simulink model "HubDepotModel"  (Simulink 7.9)
settings: Solver=VariableStepDiscrete  StartTime=0.0  StopTime=100.0  RelTol=1e-3
undefined symbols (not defined in the file or in its folder): CustomerBase_1
libraries: simeventslib x10
(part 1 of 4)
settings Model: Creator=tsprock3  LastModifiedBy=tsprock3
settings DebuggingCC: SimStateOlderReleaseMsg=warning

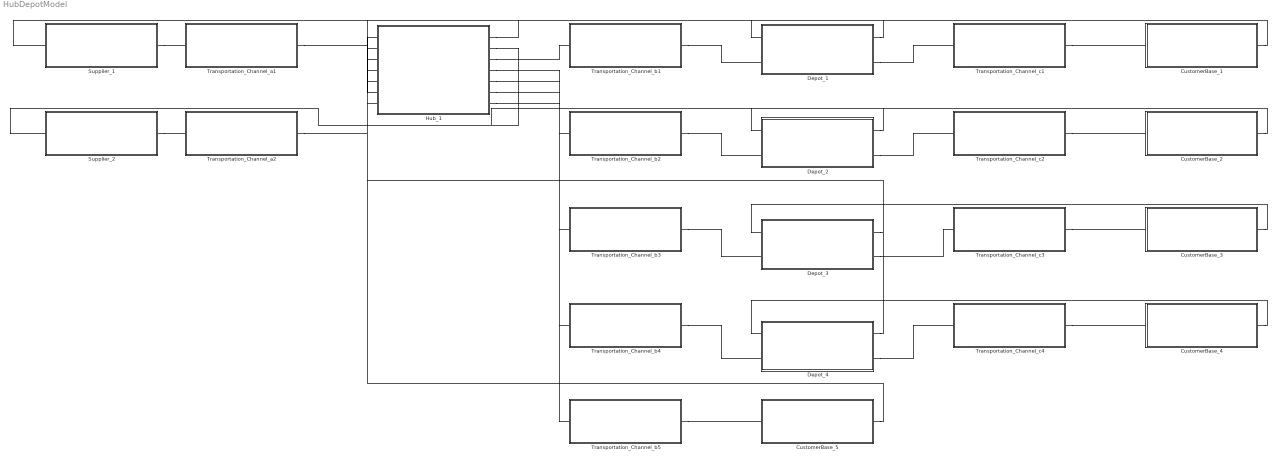
== system HubDepotModel ==
  CustomerBase_1 : Subsystem
  CustomerBase_2 : Subsystem
  CustomerBase_3 : Subsystem
  CustomerBase_4 : Subsystem
  CustomerBase_5 : Subsystem
  Depot_1 : Subsystem
  Depot_2 : Subsystem
  Depot_3 : Subsystem
  Depot_4 : Subsystem
  Hub_1 : Subsystem
  Supplier_1 : Subsystem
  Supplier_2 : Subsystem
  Transportation_Channel_a1 : Subsystem
  Transportation_Channel_a2 : Subsystem
  Transportation_Channel_b1 : Subsystem
  Transportation_Channel_b2 : Subsystem
  Transportation_Channel_b3 : Subsystem
  Transportation_Channel_b4 : Subsystem
  Transportation_Channel_b5 : Subsystem
  Transportation_Channel_c1 : Subsystem
  Transportation_Channel_c2 : Subsystem
  Transportation_Channel_c3 : Subsystem
  Transportation_Channel_c4 : Subsystem
  connections:
  CustomerBase_1/RConn1 -- Depot_1/LConn1
  CustomerBase_2/RConn1 -- Depot_2/LConn1
  CustomerBase_3/RConn1 -- Depot_3/LConn1
  CustomerBase_4/RConn1 -- Depot_4/LConn1
  CustomerBase_5/RConn1 -- Hub_1/LConn1
  Depot_1/RConn1 -- Hub_1/LConn2
  Depot_2/RConn1 -- Hub_1/LConn3
  Depot_3/RConn1 -- Hub_1/LConn4
  Depot_4/RConn1 -- Hub_1/LConn5
  Hub_1/RConn1 -- Supplier_1/LConn1
  Hub_1/RConn2 -- Supplier_2/LConn1
  Supplier_1/RConn1 -- Transportation_Channel_a1/LConn1
  Supplier_2/RConn1 -- Transportation_Channel_a2/LConn1
  Transportation_Channel_a1/RConn1 -- Hub_1/LConn6
  Transportation_Channel_a2/RConn1 -- Hub_1/LConn7
  Hub_1/RConn3 -- Transportation_Channel_b1/LConn1
  Hub_1/RConn4 -- Transportation_Channel_b2/LConn1
  Hub_1/RConn5 -- Transportation_Channel_b3/LConn1
  Hub_1/RConn6 -- Transportation_Channel_b4/LConn1
  Hub_1/RConn7 -- Transportation_Channel_b5/LConn1
  Transportation_Channel_b1/RConn1 -- Depot_1/LConn2
  Transportation_Channel_b2/RConn1 -- Depot_2/LConn2
  Transportation_Channel_b3/RConn1 -- Depot_3/LConn2
  Transportation_Channel_b4/RConn1 -- Depot_4/LConn2
  Depot_1/RConn2 -- Transportation_Channel_c1/LConn1
  Depot_2/RConn2 -- Transportation_Channel_c2/LConn1
  Depot_3/RConn2 -- Transportation_Channel_c3/LConn1
  Depot_4/RConn2 -- Transportation_Channel_c4/LConn1
  Transportation_Channel_b5/RConn1 -- CustomerBase_5/LConn1
  Transportation_Channel_c1/RConn1 -- CustomerBase_1/LConn1
  Transportation_Channel_c2/RConn1 -- CustomerBase_2/LConn1
  Transportation_Channel_c3/RConn1 -- CustomerBase_3/LConn1
  Transportation_Channel_c4/RConn1 -- CustomerBase_4/LConn1

== system HubDepotModel/CustomerBase_1 ==
  CustomerBase : Subsystem
  IN_Shipment : PathCombiner  NumberInputPorts=1
  OUT_Order : OutputSwitch  NumberOutputPorts=1  SwitchingCriterion=From attribute  AttributeName=Supplier
  IN_Shipment_1 : PMIOPort  Port=1  Side=Left
  OUT_Order_1 : PMIOPort  Port=2  Side=Right
  connections:
  IN_Shipment/RConn1 -- CustomerBase/LConn2
  OUT_Order/LConn1 -- CustomerBase/LConn1
  IN_Shipment/LConn1 -- IN_Shipment_1/RConn1
  OUT_Order/RConn1 -- OUT_Order_1/RConn1

== system HubDepotModel/CustomerBase_2 ==
  CustomerBase : Subsystem
  IN_Shipment : PathCombiner  NumberInputPorts=1
  OUT_Order : OutputSwitch  NumberOutputPorts=1  SwitchingCriterion=From attribute  AttributeName=Supplier
  IN_Shipment_1 : PMIOPort  Port=1  Side=Left
  OUT_Order_1 : PMIOPort  Port=2  Side=Right
  connections:
  IN_Shipment/RConn1 -- CustomerBase/LConn2
  OUT_Order/LConn1 -- CustomerBase/LConn1
  IN_Shipment/LConn1 -- IN_Shipment_1/RConn1
  OUT_Order/RConn1 -- OUT_Order_1/RConn1

== system HubDepotModel/CustomerBase_3 ==
  CustomerBase : Subsystem
  IN_Shipment : PathCombiner  NumberInputPorts=1
  OUT_Order : OutputSwitch  NumberOutputPorts=1  SwitchingCriterion=From attribute  AttributeName=Supplier
  IN_Shipment_1 : PMIOPort  Port=1  Side=Left
  OUT_Order_1 : PMIOPort  Port=2  Side=Right
  connections:
  IN_Shipment/RConn1 -- CustomerBase/LConn2
  OUT_Order/LConn1 -- CustomerBase/LConn1
  IN_Shipment/LConn1 -- IN_Shipment_1/RConn1
  OUT_Order/RConn1 -- OUT_Order_1/RConn1

== system HubDepotModel/CustomerBase_4 ==
  CustomerBase : Subsystem
  IN_Shipment : PathCombiner  NumberInputPorts=1
  OUT_Order : OutputSwitch  NumberOutputPorts=1  SwitchingCriterion=From attribute  AttributeName=Supplier
  IN_Shipment_1 : PMIOPort  Port=1  Side=Left
  OUT_Order_1 : PMIOPort  Port=2  Side=Right
  connections:
  IN_Shipment/RConn1 -- CustomerBase/LConn2
  OUT_Order/LConn1 -- CustomerBase/LConn1
  IN_Shipment/LConn1 -- IN_Shipment_1/RConn1
  OUT_Order/RConn1 -- OUT_Order_1/RConn1

== system HubDepotModel/CustomerBase_5 ==
  CustomerBase : Subsystem
  IN_Shipment : PathCombiner  NumberInputPorts=1
  OUT_Order : OutputSwitch  NumberOutputPorts=1  SwitchingCriterion=From attribute  AttributeName=Supplier
  IN_Shipment_1 : PMIOPort  Port=1  Side=Left
  OUT_Order_1 : PMIOPort  Port=2  Side=Right
  connections:
  IN_Shipment/RConn1 -- CustomerBase/LConn2
  OUT_Order/LConn1 -- CustomerBase/LConn1
  IN_Shipment/LConn1 -- IN_Shipment_1/RConn1
  OUT_Order/RConn1 -- OUT_Order_1/RConn1

== system HubDepotModel/Depot_1 ==
  note: IN_Order
  IN_Order : PathCombiner  NumberInputPorts=1
  IN_Shipment : PathCombiner  NumberInputPorts=1
  OUT_Order : OutputSwitch  NumberOutputPorts=1  SwitchingCriterion=From attribute  AttributeName=Supplier
  OUT_Shipment : OutputSwitch  NumberOutputPorts=1  SwitchingCriterion=From attribute  AttributeName=Customer
  Storage_Subsystem : Subsystem
  IN_Order_1 : PMIOPort  Port=1  Side=Left
  IN_Shipment_1 : PMIOPort  Port=2  Side=Left
  OUT_Order_1 : PMIOPort  Port=3  Side=Right
  OUT_Shipment_1 : PMIOPort  Port=4  Side=Right
  connections:
  Storage_Subsystem/RConn2 -- OUT_Shipment/LConn1
  IN_Order/RConn1 -- Storage_Subsystem/RConn1
  OUT_Order/LConn1 -- Storage_Subsystem/LConn1
  IN_Shipment/RConn1 -- Storage_Subsystem/LConn2
  IN_Order/LConn1 -- IN_Order_1/RConn1
  IN_Shipment/LConn1 -- IN_Shipment_1/RConn1
  OUT_Order/RConn1 -- OUT_Order_1/RConn1
  OUT_Shipment/RConn1 -- OUT_Shipment_1/RConn1

== system HubDepotModel/Depot_2 ==
  note: IN_Order
  IN_Order : PathCombiner  NumberInputPorts=1
  IN_Shipment : PathCombiner  NumberInputPorts=1
  OUT_Order : OutputSwitch  NumberOutputPorts=1  SwitchingCriterion=From attribute  AttributeName=Supplier
  OUT_Shipment : OutputSwitch  NumberOutputPorts=1  SwitchingCriterion=From attribute  AttributeName=Customer
  Storage_Subsystem : Subsystem
  IN_Order_1 : PMIOPort  Port=1  Side=Left
  IN_Shipment_1 : PMIOPort  Port=2  Side=Left
  OUT_Order_1 : PMIOPort  Port=3  Side=Right
  OUT_Shipment_1 : PMIOPort  Port=4  Side=Right
  connections:
  Storage_Subsystem/RConn2 -- OUT_Shipment/LConn1
  IN_Order/RConn1 -- Storage_Subsystem/RConn1
  OUT_Order/LConn1 -- Storage_Subsystem/LConn1
  IN_Shipment/RConn1 -- Storage_Subsystem/LConn2
  IN_Order/LConn1 -- IN_Order_1/RConn1
  IN_Shipment/LConn1 -- IN_Shipment_1/RConn1
  OUT_Order/RConn1 -- OUT_Order_1/RConn1
  OUT_Shipment/RConn1 -- OUT_Shipment_1/RConn1

== system HubDepotModel/Depot_3 ==
  note: IN_Order
  IN_Order : PathCombiner  NumberInputPorts=1
  IN_Shipment : PathCombiner  NumberInputPorts=1
  OUT_Order : OutputSwitch  NumberOutputPorts=1  SwitchingCriterion=From attribute  AttributeName=Supplier
  OUT_Shipment : OutputSwitch  NumberOutputPorts=1  SwitchingCriterion=From attribute  AttributeName=Customer
  Storage_Subsystem : Subsystem
  IN_Order_1 : PMIOPort  Port=1  Side=Left
  IN_Shipment_1 : PMIOPort  Port=2  Side=Left
  OUT_Order_1 : PMIOPort  Port=3  Side=Right
  OUT_Shipment_1 : PMIOPort  Port=4  Side=Right
  connections:
  Storage_Subsystem/RConn2 -- OUT_Shipment/LConn1
  IN_Order/RConn1 -- Storage_Subsystem/RConn1
  OUT_Order/LConn1 -- Storage_Subsystem/LConn1
  IN_Shipment/RConn1 -- Storage_Subsystem/LConn2
  IN_Order/LConn1 -- IN_Order_1/RConn1
  IN_Shipment/LConn1 -- IN_Shipment_1/RConn1
  OUT_Order/RConn1 -- OUT_Order_1/RConn1
  OUT_Shipment/RConn1 -- OUT_Shipment_1/RConn1

== system HubDepotModel/Depot_4 ==
  note: IN_Order
  IN_Order : PathCombiner  NumberInputPorts=1
  IN_Shipment : PathCombiner  NumberInputPorts=1
  OUT_Order : OutputSwitch  NumberOutputPorts=1  SwitchingCriterion=From attribute  AttributeName=Supplier
  OUT_Shipment : OutputSwitch  NumberOutputPorts=1  SwitchingCriterion=From attribute  AttributeName=Customer
  Storage_Subsystem : Subsystem
  IN_Order_1 : PMIOPort  Port=1  Side=Left
  IN_Shipment_1 : PMIOPort  Port=2  Side=Left
  OUT_Order_1 : PMIOPort  Port=3  Side=Right
  OUT_Shipment_1 : PMIOPort  Port=4  Side=Right
  connections:
  Storage_Subsystem/RConn2 -- OUT_Shipment/LConn1
  IN_Order/RConn1 -- Storage_Subsystem/RConn1
  OUT_Order/LConn1 -- Storage_Subsystem/LConn1
  IN_Shipment/RConn1 -- Storage_Subsystem/LConn2
  IN_Order/LConn1 -- IN_Order_1/RConn1
  IN_Shipment/LConn1 -- IN_Shipment_1/RConn1
  OUT_Order/RConn1 -- OUT_Order_1/RConn1
  OUT_Shipment/RConn1 -- OUT_Shipment_1/RConn1

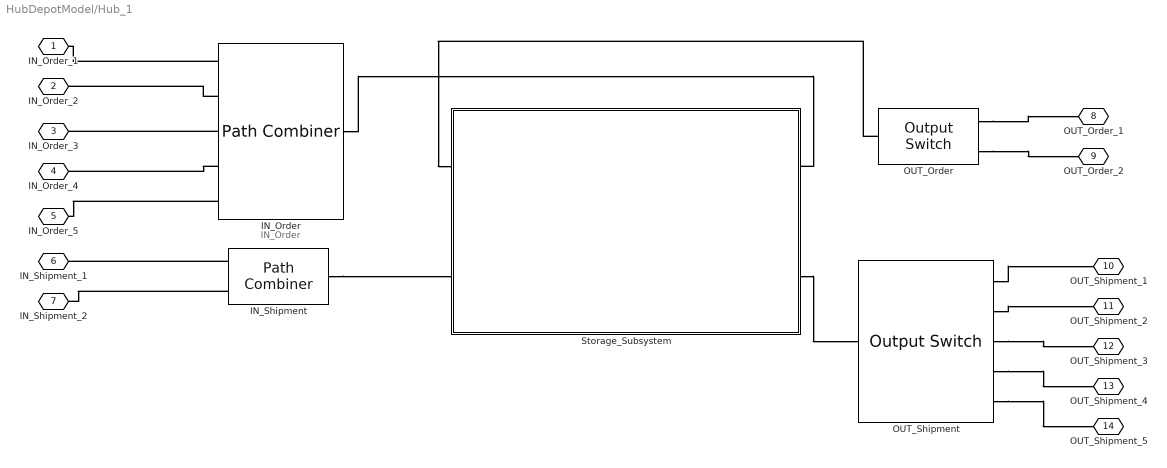
== system HubDepotModel/Hub_1 ==
  note: IN_Order
  IN_Order : PathCombiner  NumberInputPorts=5
  IN_Shipment : PathCombiner  NumberInputPorts=2
  OUT_Order : OutputSwitch  NumberOutputPorts=2  SwitchingCriterion=From attribute  AttributeName=Supplier
  OUT_Shipment : OutputSwitch  NumberOutputPorts=5  SwitchingCriterion=From attribute  AttributeName=Customer
  Storage_Subsystem : Subsystem
  IN_Order_1 : PMIOPort  Port=1  Side=Left
  IN_Order_2 : PMIOPort  Port=2  Side=Left
  IN_Order_3 : PMIOPort  Port=3  Side=Left
  IN_Order_4 : PMIOPort  Port=4  Side=Left
  IN_Order_5 : PMIOPort  Port=5  Side=Left
  IN_Shipment_1 : PMIOPort  Port=6  Side=Left
  IN_Shipment_2 : PMIOPort  Port=7  Side=Left
  OUT_Order_1 : PMIOPort  Port=8  Side=Right
  OUT_Order_2 : PMIOPort  Port=9  Side=Right
  OUT_Shipment_1 : PMIOPort  Port=10  Side=Right
  OUT_Shipment_2 : PMIOPort  Port=11  Side=Right
  OUT_Shipment_3 : PMIOPort  Port=12  Side=Right
  OUT_Shipment_4 : PMIOPort  Port=13  Side=Right
  OUT_Shipment_5 : PMIOPort  Port=14  Side=Right
  connections:
  Storage_Subsystem/RConn2 -- OUT_Shipment/LConn1
  IN_Order/RConn1 -- Storage_Subsystem/RConn1
  OUT_Order/LConn1 -- Storage_Subsystem/LConn1
  IN_Shipment/RConn1 -- Storage_Subsystem/LConn2
  IN_Order/LConn1 -- IN_Order_1/RConn1
  IN_Order/LConn2 -- IN_Order_2/RConn1
  IN_Order/LConn3 -- IN_Order_3/RConn1
  IN_Order/LConn4 -- IN_Order_4/RConn1
  IN_Order/LConn5 -- IN_Order_5/RConn1
  IN_Shipment/LConn1 -- IN_Shipment_1/RConn1
  IN_Shipment/LConn2 -- IN_Shipment_2/RConn1
  OUT_Order/RConn1 -- OUT_Order_1/RConn1
  OUT_Order/RConn2 -- OUT_Order_2/RConn1
  OUT_Shipment/RConn1 -- OUT_Shipment_1/RConn1
  OUT_Shipment/RConn2 -- OUT_Shipment_2/RConn1
  OUT_Shipment/RConn3 -- OUT_Shipment_3/RConn1
  OUT_Shipment/RConn4 -- OUT_Shipment_4/RConn1
  OUT_Shipment/RConn5 -- OUT_Shipment_5/RConn1

== system HubDepotModel/Supplier_1 ==
  IN_Order : PathCombiner  NumberInputPorts=1
  OUT_Shipment : OutputSwitch  NumberOutputPorts=1  SwitchingCriterion=From attribute  AttributeName=Customer
  Supplier : Subsystem
  IN_Order_1 : PMIOPort  Port=1  Side=Left
  OUT_Shipment_1 : PMIOPort  Port=2  Side=Right
  connections:
  IN_Order/RConn1 -- Supplier/RConn2
  OUT_Shipment/LConn1 -- Supplier/RConn1
  IN_Order/LConn1 -- IN_Order_1/RConn1
  OUT_Shipment/RConn1 -- OUT_Shipment_1/RConn1

== system HubDepotModel/Supplier_2 ==
  IN_Order : PathCombiner  NumberInputPorts=1
  OUT_Shipment : OutputSwitch  NumberOutputPorts=1  SwitchingCriterion=From attribute  AttributeName=Customer
  Supplier : Subsystem
  IN_Order_1 : PMIOPort  Port=1  Side=Left
  OUT_Shipment_1 : PMIOPort  Port=2  Side=Right
  connections:
  IN_Order/RConn1 -- Supplier/RConn2
  OUT_Shipment/LConn1 -- Supplier/RConn1
  IN_Order/LConn1 -- IN_Order_1/RConn1
  OUT_Shipment/RConn1 -- OUT_Shipment_1/RConn1

== system HubDepotModel/Transportation_Channel_a1 ==
  FIFO Queue : FIFOQueue  Capacity=inf
  IN_Shipment : PathCombiner  NumberInputPorts=1
  N-Server : NServer  NumberOfServers=inf  ServiceTime=0
  OUT_Shipment : OutputSwitch  NumberOutputPorts=1  AttributeName=Customer
  IN_Shipment_1 : PMIOPort  Port=1  Side=Left
  OUT_Shipment_1 : PMIOPort  Port=2  Side=Right
  connections:
  N-Server/RConn1 -- OUT_Shipment/LConn1
  IN_Shipment/RConn1 -- FIFO Queue/LConn1
  FIFO Queue/RConn1 -- N-Server/LConn1
  IN_Shipment/LConn1 -- IN_Shipment_1/RConn1
  OUT_Shipment/RConn1 -- OUT_Shipment_1/RConn1

== system HubDepotModel/Transportation_Channel_a2 ==
  FIFO Queue : FIFOQueue  Capacity=inf
  IN_Shipment : PathCombiner  NumberInputPorts=1
  N-Server : NServer  NumberOfServers=inf  ServiceTime=0
  OUT_Shipment : OutputSwitch  NumberOutputPorts=1  AttributeName=Customer
  IN_Shipment_1 : PMIOPort  Port=1  Side=Left
  OUT_Shipment_1 : PMIOPort  Port=2  Side=Right
  connections:
  N-Server/RConn1 -- OUT_Shipment/LConn1
  IN_Shipment/RConn1 -- FIFO Queue/LConn1
  FIFO Queue/RConn1 -- N-Server/LConn1
  IN_Shipment/LConn1 -- IN_Shipment_1/RConn1
  OUT_Shipment/RConn1 -- OUT_Shipment_1/RConn1

== system HubDepotModel/Transportation_Channel_b1 ==
  FIFO Queue : FIFOQueue  Capacity=inf
  IN_Shipment : PathCombiner  NumberInputPorts=1
  N-Server : NServer  NumberOfServers=inf  ServiceTime=0
  OUT_Shipment : OutputSwitch  NumberOutputPorts=1  AttributeName=Customer
  IN_Shipment_1 : PMIOPort  Port=1  Side=Left
  OUT_Shipment_1 : PMIOPort  Port=2  Side=Right
  connections:
  N-Server/RConn1 -- OUT_Shipment/LConn1
  IN_Shipment/RConn1 -- FIFO Queue/LConn1
  FIFO Queue/RConn1 -- N-Server/LConn1
  IN_Shipment/LConn1 -- IN_Shipment_1/RConn1
  OUT_Shipment/RConn1 -- OUT_Shipment_1/RConn1

== system HubDepotModel/Transportation_Channel_b2 ==
  FIFO Queue : FIFOQueue  Capacity=inf
  IN_Shipment : PathCombiner  NumberInputPorts=1
  N-Server : NServer  NumberOfServers=inf  ServiceTime=0
  OUT_Shipment : OutputSwitch  NumberOutputPorts=1  AttributeName=Customer
  IN_Shipment_1 : PMIOPort  Port=1  Side=Left
  OUT_Shipment_1 : PMIOPort  Port=2  Side=Right
  connections:
  N-Server/RConn1 -- OUT_Shipment/LConn1
  IN_Shipment/RConn1 -- FIFO Queue/LConn1
  FIFO Queue/RConn1 -- N-Server/LConn1
  IN_Shipment/LConn1 -- IN_Shipment_1/RConn1
  OUT_Shipment/RConn1 -- OUT_Shipment_1/RConn1

== system HubDepotModel/Transportation_Channel_b3 ==
  FIFO Queue : FIFOQueue  Capacity=inf
  IN_Shipment : PathCombiner  NumberInputPorts=1
  N-Server : NServer  NumberOfServers=inf  ServiceTime=0
  OUT_Shipment : OutputSwitch  NumberOutputPorts=1  AttributeName=Customer
  IN_Shipment_1 : PMIOPort  Port=1  Side=Left
  OUT_Shipment_1 : PMIOPort  Port=2  Side=Right
  connections:
  N-Server/RConn1 -- OUT_Shipment/LConn1
  IN_Shipment/RConn1 -- FIFO Queue/LConn1
  FIFO Queue/RConn1 -- N-Server/LConn1
  IN_Shipment/LConn1 -- IN_Shipment_1/RConn1
  OUT_Shipment/RConn1 -- OUT_Shipment_1/RConn1

== system HubDepotModel/Transportation_Channel_b4 ==
  FIFO Queue : FIFOQueue  Capacity=inf
  IN_Shipment : PathCombiner  NumberInputPorts=1
  N-Server : NServer  NumberOfServers=inf  ServiceTime=0
  OUT_Shipment : OutputSwitch  NumberOutputPorts=1  AttributeName=Customer
  IN_Shipment_1 : PMIOPort  Port=1  Side=Left
  OUT_Shipment_1 : PMIOPort  Port=2  Side=Right
  connections:
  N-Server/RConn1 -- OUT_Shipment/LConn1
  IN_Shipment/RConn1 -- FIFO Queue/LConn1
  FIFO Queue/RConn1 -- N-Server/LConn1
  IN_Shipment/LConn1 -- IN_Shipment_1/RConn1
  OUT_Shipment/RConn1 -- OUT_Shipment_1/RConn1

== system HubDepotModel/Transportation_Channel_b5 ==
  FIFO Queue : FIFOQueue  Capacity=inf
  IN_Shipment : PathCombiner  NumberInputPorts=1
  N-Server : NServer  NumberOfServers=inf  ServiceTime=0
  OUT_Shipment : OutputSwitch  NumberOutputPorts=1  AttributeName=Customer
  IN_Shipment_1 : PMIOPort  Port=1  Side=Left
  OUT_Shipment_1 : PMIOPort  Port=2  Side=Right
  connections:
  N-Server/RConn1 -- OUT_Shipment/LConn1
  IN_Shipment/RConn1 -- FIFO Queue/LConn1
  FIFO Queue/RConn1 -- N-Server/LConn1
  IN_Shipment/LConn1 -- IN_Shipment_1/RConn1
  OUT_Shipment/RConn1 -- OUT_Shipment_1/RConn1

== system HubDepotModel/Transportation_Channel_c1 ==
  FIFO Queue : FIFOQueue  Capacity=inf
  IN_Shipment : PathCombiner  NumberInputPorts=1
  N-Server : NServer  NumberOfServers=inf  ServiceTime=0
  OUT_Shipment : OutputSwitch  NumberOutputPorts=1  AttributeName=Customer
  IN_Shipment_1 : PMIOPort  Port=1  Side=Left
  OUT_Shipment_1 : PMIOPort  Port=2  Side=Right
  connections:
  N-Server/RConn1 -- OUT_Shipment/LConn1
  IN_Shipment/RConn1 -- FIFO Queue/LConn1
  FIFO Queue/RConn1 -- N-Server/LConn1
  IN_Shipment/LConn1 -- IN_Shipment_1/RConn1
  OUT_Shipment/RConn1 -- OUT_Shipment_1/RConn1

== system HubDepotModel/Transportation_Channel_c2 ==
  FIFO Queue : FIFOQueue  Capacity=inf
  IN_Shipment : PathCombiner  NumberInputPorts=1
  N-Server : NServer  NumberOfServers=inf  ServiceTime=0
  OUT_Shipment : OutputSwitch  NumberOutputPorts=1  AttributeName=Customer
  IN_Shipment_1 : PMIOPort  Port=1  Side=Left
  OUT_Shipment_1 : PMIOPort  Port=2  Side=Right
  connections:
  N-Server/RConn1 -- OUT_Shipment/LConn1
  IN_Shipment/RConn1 -- FIFO Queue/LConn1
  FIFO Queue/RConn1 -- N-Server/LConn1
  IN_Shipment/LConn1 -- IN_Shipment_1/RConn1
  OUT_Shipment/RConn1 -- OUT_Shipment_1/RConn1

== system HubDepotModel/Transportation_Channel_c3 ==
  FIFO Queue : FIFOQueue  Capacity=inf
  IN_Shipment : PathCombiner  NumberInputPorts=1
  N-Server : NServer  NumberOfServers=inf  ServiceTime=0
  OUT_Shipment : OutputSwitch  NumberOutputPorts=1  AttributeName=Customer
  IN_Shipment_1 : PMIOPort  Port=1  Side=Left
  OUT_Shipment_1 : PMIOPort  Port=2  Side=Right
  connections:
  N-Server/RConn1 -- OUT_Shipment/LConn1
  IN_Shipment/RConn1 -- FIFO Queue/LConn1
  FIFO Queue/RConn1 -- N-Server/LConn1
  IN_Shipment/LConn1 -- IN_Shipment_1/RConn1
  OUT_Shipment/RConn1 -- OUT_Shipment_1/RConn1

== system HubDepotModel/Transportation_Channel_c4 ==
  FIFO Queue : FIFOQueue  Capacity=inf
  IN_Shipment : PathCombiner  NumberInputPorts=1
  N-Server : NServer  NumberOfServers=inf  ServiceTime=0
  OUT_Shipment : OutputSwitch  NumberOutputPorts=1  AttributeName=Customer
  IN_Shipment_1 : PMIOPort  Port=1  Side=Left
  OUT_Shipment_1 : PMIOPort  Port=2  Side=Right
  connections:
  N-Server/RConn1 -- OUT_Shipment/LConn1
  IN_Shipment/RConn1 -- FIFO Queue/LConn1
  FIFO Queue/RConn1 -- N-Server/LConn1
  IN_Shipment/LConn1 -- IN_Shipment_1/RConn1
  OUT_Shipment/RConn1 -- OUT_Shipment_1/RConn1

== system HubDepotModel/CustomerBase_1/CustomerBase ==
  Consumption_Component : EventBasedSequence  VectorOutputValues=CustomerBase_1(:,1)
  Entity Sink : EntitySink
  Order_Generator : TimeBasedEntityGenerator  GenerateEntitiesUpon=Intergeneration time from port t  GenerateEntityAtSimulationStart=off
  Order_Quantity : EventBasedSequence  VectorOutputValues=CustomerBase_1(:,2)
  Order_Time : EventBasedSequence  VectorOutputValues=CustomerBase_1(:,3)  FormOutputOpt=Setting to infinity
  Set_Procurement_Order : SetAttribute  AttributeName=Component|Order_Quantity|Customer|Supplier  AttributeFrom=Signal port|Signal port|Dialog|Dialog  AttributeValue=1|3|1|1  AttributeTreatAsVector=1|1|1|1  EvaluatedAttributeValue={[];[];1;1}
      settings: InputPortMap=u0,u1
  Procurement_Order : PMIOPort  Port=1  Side=Left
  Replenishment_Shipment : PMIOPort  Port=2  Side=Left
  wires:
  Consumption_Component/1 -> Set_Procurement_Order/1
  Order_Quantity/1 -> Set_Procurement_Order/2
  Order_Time/1 -> Order_Generator/1
  connections:
  Replenishment_Shipment/RConn1 -- Entity Sink/LConn1
  Procurement_Order/RConn1 -- Set_Procurement_Order/RConn1
  Order_Generator/RConn1 -- Set_Procurement_Order/LConn1

== system HubDepotModel/CustomerBase_2/CustomerBase ==
  Consumption_Component : EventBasedSequence  VectorOutputValues=[2 1 2 1 2 1].'
  Entity Sink : EntitySink
  Order_Generator : TimeBasedEntityGenerator  GenerateEntitiesUpon=Intergeneration time from port t  GenerateEntityAtSimulationStart=off
  Order_Quantity : EventBasedRandomNumber  Distribution=Arbitrary discrete  valueVecDisc=[1 2 3 4 5]  probVecDisc=[0.2 0.2 0.2 0.2 0.2]  Seed=46469
  Order_Time : EventBasedSequence  VectorOutputValues=[0; 0; 1; 0; 1; 1; 1; 0; 0; 1; 1; 0; 1].'
  Set_Procurement_Order : SetAttribute  AttributeName=Component|Order_Quantity|Customer|Supplier  AttributeFrom=Signal port|Signal port|Dialog|Dialog  AttributeValue=1|3|1|1  AttributeTreatAsVector=1|1|1|1  EvaluatedAttributeValue={[];[];1;1}
      settings: InputPortMap=u0,u1
  Procurement_Order : PMIOPort  Port=1  Side=Left
  Replenishment_Shipment : PMIOPort  Port=2  Side=Left
  wires:
  Consumption_Component/1 -> Set_Procurement_Order/1
  Order_Quantity/1 -> Set_Procurement_Order/2
  Order_Time/1 -> Order_Generator/1
  connections:
  Replenishment_Shipment/RConn1 -- Entity Sink/LConn1
  Procurement_Order/RConn1 -- Set_Procurement_Order/RConn1
  Order_Generator/RConn1 -- Set_Procurement_Order/LConn1

== system HubDepotModel/CustomerBase_3/CustomerBase ==
  Consumption_Component : EventBasedSequence  VectorOutputValues=[2 1 2 1 2 1].'
  Entity Sink : EntitySink
  Order_Generator : TimeBasedEntityGenerator  GenerateEntitiesUpon=Intergeneration time from port t  GenerateEntityAtSimulationStart=off
  Order_Quantity : EventBasedRandomNumber  Distribution=Arbitrary discrete  valueVecDisc=[1 2 3 4 5]  probVecDisc=[0.2 0.2 0.2 0.2 0.2]  Seed=1431
  Order_Time : EventBasedSequence  VectorOutputValues=[0; 0; 1; 0; 1; 1; 1; 0; 0; 1; 1; 0; 1].'
  Set_Procurement_Order : SetAttribute  AttributeName=Component|Order_Quantity|Customer|Supplier  AttributeFrom=Signal port|Signal port|Dialog|Dialog  AttributeValue=1|3|1|1  AttributeTreatAsVector=1|1|1|1  EvaluatedAttributeValue={[];[];1;1}
      settings: InputPortMap=u0,u1
  Procurement_Order : PMIOPort  Port=1  Side=Left
  Replenishment_Shipment : PMIOPort  Port=2  Side=Left
  wires:
  Consumption_Component/1 -> Set_Procurement_Order/1
  Order_Quantity/1 -> Set_Procurement_Order/2
  Order_Time/1 -> Order_Generator/1
  connections:
  Replenishment_Shipment/RConn1 -- Entity Sink/LConn1
  Procurement_Order/RConn1 -- Set_Procurement_Order/RConn1
  Order_Generator/RConn1 -- Set_Procurement_Order/LConn1

== system HubDepotModel/CustomerBase_4/CustomerBase ==
  Consumption_Component : EventBasedSequence  VectorOutputValues=[2 1 2 1 2 1].'
  Entity Sink : EntitySink
  Order_Generator : TimeBasedEntityGenerator  GenerateEntitiesUpon=Intergeneration time from port t  GenerateEntityAtSimulationStart=off
  Order_Quantity : EventBasedRandomNumber  Distribution=Arbitrary discrete  valueVecDisc=[1 2 3 4 5]  probVecDisc=[0.2 0.2 0.2 0.2 0.2]  Seed=4648
  Order_Time : EventBasedSequence  VectorOutputValues=[0; 0; 1; 0; 1; 1; 1; 0; 0; 1; 1; 0; 1].'
  Set_Procurement_Order : SetAttribute  AttributeName=Component|Order_Quantity|Customer|Supplier  AttributeFrom=Signal port|Signal port|Dialog|Dialog  AttributeValue=1|3|1|1  AttributeTreatAsVector=1|1|1|1  EvaluatedAttributeValue={[];[];1;1}
      settings: InputPortMap=u0,u1
  Procurement_Order : PMIOPort  Port=1  Side=Left
  Replenishment_Shipment : PMIOPort  Port=2  Side=Left
  wires:
  Consumption_Component/1 -> Set_Procurement_Order/1
  Order_Quantity/1 -> Set_Procurement_Order/2
  Order_Time/1 -> Order_Generator/1
  connections:
  Replenishment_Shipment/RConn1 -- Entity Sink/LConn1
  Procurement_Order/RConn1 -- Set_Procurement_Order/RConn1
  Order_Generator/RConn1 -- Set_Procurement_Order/LConn1

== system HubDepotModel/CustomerBase_5/CustomerBase ==
  Consumption_Component : EventBasedSequence  VectorOutputValues=[2 1 2 1 2 1].'
  Entity Sink : EntitySink
  Order_Generator : TimeBasedEntityGenerator  GenerateEntitiesUpon=Intergeneration time from port t  GenerateEntityAtSimulationStart=off
  Order_Quantity : EventBasedRandomNumber  Distribution=Arbitrary discrete  valueVecDisc=[1 2 3 4 5]  probVecDisc=[0.2 0.2 0.2 0.2 0.2]  Seed=7865
  Order_Time : EventBasedSequence  VectorOutputValues=[0; 0; 1; 0; 1; 1; 1; 0; 0; 1; 1; 0; 1].'
  Set_Procurement_Order : SetAttribute  AttributeName=Component|Order_Quantity|Customer|Supplier  AttributeFrom=Signal port|Signal port|Dialog|Dialog  AttributeValue=1|3|1|1  AttributeTreatAsVector=1|1|1|1  EvaluatedAttributeValue={[];[];1;1}
      settings: InputPortMap=u0,u1
  Procurement_Order : PMIOPort  Port=1  Side=Left
  Replenishment_Shipment : PMIOPort  Port=2  Side=Left
  wires:
  Consumption_Component/1 -> Set_Procurement_Order/1
  Order_Quantity/1 -> Set_Procurement_Order/2
  Order_Time/1 -> Order_Generator/1
  connections:
  Replenishment_Shipment/RConn1 -- Entity Sink/LConn1
  Procurement_Order/RConn1 -- Set_Procurement_Order/RConn1
  Order_Generator/RConn1 -- Set_Procurement_Order/LConn1

== system HubDepotModel/Depot_1/Storage_Subsystem ==
  <<DELIVER>>Deliver_Stocked_Product : Subsystem
  <<ENABLE>> Manage_Product_Inventory : Subsystem
  <<SOURCE>> Source_Stocked_Product : Subsystem
  Customer_Procurement_Order : PMIOPort  Port=1  Side=Right
  Fulfillment_Shipment : PMIOPort  Port=2  Side=Right
  Procurement_Order : PMIOPort  Port=3  Side=Left
  Replenishment_Shipment : PMIOPort  Port=4  Side=Left
  connections:
  <<DELIVER>>Deliver_Stocked_Product/RConn1 -- <<ENABLE>> Manage_Product_Inventory/LConn1
  <<SOURCE>> Source_Stocked_Product/RConn2 -- Procurement_Order/RConn1
  <<ENABLE>> Manage_Product_Inventory/RConn3 -- <<SOURCE>> Source_Stocked_Product/LConn3
  <<ENABLE>> Manage_Product_Inventory/LConn3 -- <<DELIVER>>Deliver_Stocked_Product/RConn3
  <<ENABLE>> Manage_Product_Inventory/RConn2 -- <<SOURCE>> Source_Stocked_Product/LConn1
  <<ENABLE>> Manage_Product_Inventory/LConn2 -- <<SOURCE>> Source_Stocked_Product/RConn1
  Replenishment_Shipment/RConn1 -- <<SOURCE>> Source_Stocked_Product/LConn2
  <<DELIVER>>Deliver_Stocked_Product/RConn2 -- Fulfillment_Shipment/RConn1
  <<DELIVER>>Deliver_Stocked_Product/LConn2 -- Customer_Procurement_Order/RConn1
  <<DELIVER>>Deliver_Stocked_Product/LConn1 -- <<ENABLE>> Manage_Product_Inventory/RConn1

== system HubDepotModel/Depot_2/Storage_Subsystem ==
  <<DELIVER>>Deliver_Stocked_Product : Subsystem
  <<ENABLE>> Manage_Product_Inventory : Subsystem
  <<SOURCE>> Source_Stocked_Product : Subsystem
  Customer_Procurement_Order : PMIOPort  Port=1  Side=Right
  Fulfillment_Shipment : PMIOPort  Port=2  Side=Right
  Procurement_Order : PMIOPort  Port=3  Side=Left
  Replenishment_Shipment : PMIOPort  Port=4  Side=Left
  connections:
  <<DELIVER>>Deliver_Stocked_Product/RConn1 -- <<ENABLE>> Manage_Product_Inventory/LConn1
  <<SOURCE>> Source_Stocked_Product/RConn2 -- Procurement_Order/RConn1
  <<ENABLE>> Manage_Product_Inventory/RConn3 -- <<SOURCE>> Source_Stocked_Product/LConn3
  <<ENABLE>> Manage_Product_Inventory/LConn3 -- <<DELIVER>>Deliver_Stocked_Product/RConn3
  <<ENABLE>> Manage_Product_Inventory/RConn2 -- <<SOURCE>> Source_Stocked_Product/LConn1
  <<ENABLE>> Manage_Product_Inventory/LConn2 -- <<SOURCE>> Source_Stocked_Product/RConn1
  Replenishment_Shipment/RConn1 -- <<SOURCE>> Source_Stocked_Product/LConn2
  <<DELIVER>>Deliver_Stocked_Product/RConn2 -- Fulfillment_Shipment/RConn1
  <<DELIVER>>Deliver_Stocked_Product/LConn2 -- Customer_Procurement_Order/RConn1
  <<DELIVER>>Deliver_Stocked_Product/LConn1 -- <<ENABLE>> Manage_Product_Inventory/RConn1

== system HubDepotModel/Depot_3/Storage_Subsystem ==
  <<DELIVER>>Deliver_Stocked_Product : Subsystem
  <<ENABLE>> Manage_Product_Inventory : Subsystem
  <<SOURCE>> Source_Stocked_Product : Subsystem
  Customer_Procurement_Order : PMIOPort  Port=1  Side=Right
  Fulfillment_Shipment : PMIOPort  Port=2  Side=Right
  Procurement_Order : PMIOPort  Port=3  Side=Left
  Replenishment_Shipment : PMIOPort  Port=4  Side=Left
  connections:
  <<DELIVER>>Deliver_Stocked_Product/RConn1 -- <<ENABLE>> Manage_Product_Inventory/LConn1
  <<SOURCE>> Source_Stocked_Product/RConn2 -- Procurement_Order/RConn1
  <<ENABLE>> Manage_Product_Inventory/RConn3 -- <<SOURCE>> Source_Stocked_Product/LConn3
  <<ENABLE>> Manage_Product_Inventory/LConn3 -- <<DELIVER>>Deliver_Stocked_Product/RConn3
  <<ENABLE>> Manage_Product_Inventory/RConn2 -- <<SOURCE>> Source_Stocked_Product/LConn1
  <<ENABLE>> Manage_Product_Inventory/LConn2 -- <<SOURCE>> Source_Stocked_Product/RConn1
  Replenishment_Shipment/RConn1 -- <<SOURCE>> Source_Stocked_Product/LConn2
  <<DELIVER>>Deliver_Stocked_Product/RConn2 -- Fulfillment_Shipment/RConn1
  <<DELIVER>>Deliver_Stocked_Product/LConn2 -- Customer_Procurement_Order/RConn1
  <<DELIVER>>Deliver_Stocked_Product/LConn1 -- <<ENABLE>> Manage_Product_Inventory/RConn1

== system HubDepotModel/Depot_4/Storage_Subsystem ==
  <<DELIVER>>Deliver_Stocked_Product : Subsystem
  <<ENABLE>> Manage_Product_Inventory : Subsystem
  <<SOURCE>> Source_Stocked_Product : Subsystem
  Customer_Procurement_Order : PMIOPort  Port=1  Side=Right
  Fulfillment_Shipment : PMIOPort  Port=2  Side=Right
  Procurement_Order : PMIOPort  Port=3  Side=Left
  Replenishment_Shipment : PMIOPort  Port=4  Side=Left
  connections:
  <<DELIVER>>Deliver_Stocked_Product/RConn1 -- <<ENABLE>> Manage_Product_Inventory/LConn1
  <<SOURCE>> Source_Stocked_Product/RConn2 -- Procurement_Order/RConn1
  <<ENABLE>> Manage_Product_Inventory/RConn3 -- <<SOURCE>> Source_Stocked_Product/LConn3
  <<ENABLE>> Manage_Product_Inventory/LConn3 -- <<DELIVER>>Deliver_Stocked_Product/RConn3
  <<ENABLE>> Manage_Product_Inventory/RConn2 -- <<SOURCE>> Source_Stocked_Product/LConn1
  <<ENABLE>> Manage_Product_Inventory/LConn2 -- <<SOURCE>> Source_Stocked_Product/RConn1
  Replenishment_Shipment/RConn1 -- <<SOURCE>> Source_Stocked_Product/LConn2
  <<DELIVER>>Deliver_Stocked_Product/RConn2 -- Fulfillment_Shipment/RConn1
  <<DELIVER>>Deliver_Stocked_Product/LConn2 -- Customer_Procurement_Order/RConn1
  <<DELIVER>>Deliver_Stocked_Product/LConn1 -- <<ENABLE>> Manage_Product_Inventory/RConn1

== system HubDepotModel/Hub_1/Storage_Subsystem ==
  <<DELIVER>>Deliver_Stocked_Product : Subsystem
  <<ENABLE>> Manage_Product_Inventory : Subsystem
  <<SOURCE>> Source_Stocked_Product : Subsystem
  Customer_Procurement_Order : PMIOPort  Port=1  Side=Right
  Fulfillment_Shipment : PMIOPort  Port=2  Side=Right
  Procurement_Order : PMIOPort  Port=3  Side=Left
  Replenishment_Shipment : PMIOPort  Port=4  Side=Left
  connections:
  <<DELIVER>>Deliver_Stocked_Product/RConn1 -- <<ENABLE>> Manage_Product_Inventory/LConn1
  <<SOURCE>> Source_Stocked_Product/RConn2 -- Procurement_Order/RConn1
  <<ENABLE>> Manage_Product_Inventory/RConn3 -- <<SOURCE>> Source_Stocked_Product/LConn3
  <<ENABLE>> Manage_Product_Inventory/LConn3 -- <<DELIVER>>Deliver_Stocked_Product/RConn3
  <<ENABLE>> Manage_Product_Inventory/RConn2 -- <<SOURCE>> Source_Stocked_Product/LConn1
  <<ENABLE>> Manage_Product_Inventory/LConn2 -- <<SOURCE>> Source_Stocked_Product/RConn1
  Replenishment_Shipment/RConn1 -- <<SOURCE>> Source_Stocked_Product/LConn2
  <<DELIVER>>Deliver_Stocked_Product/RConn2 -- Fulfillment_Shipment/RConn1
  <<DELIVER>>Deliver_Stocked_Product/LConn2 -- Customer_Procurement_Order/RConn1
  <<DELIVER>>Deliver_Stocked_Product/LConn1 -- <<ENABLE>> Manage_Product_Inventory/RConn1

== system HubDepotModel/Supplier_1/Supplier ==
  FIFO Queue : FIFOQueue
  Get_Order_Attributes : GetAttribute  AttributeName=Order_Quantity|Component  AttributeMissing=Error|Error  AttributeDefaultValue=1|1  AttributeTreatAsVector=1|1  AttributeSendTiming=After entity departure|After entity departure  EvaluatedDefaultAttributeValue={[];[]}
      settings: OutputPortMap=o1,o2
  N-Server : NServer  NumberOfServers=inf  ServiceTime=0
  Set_Shipment_Attributes : SetAttribute  AttributeName=Component|Shipment_Quantity  AttributeFrom=Signal port|Signal port  AttributeValue=1|3  AttributeTreatAsVector=1|1  EvaluatedAttributeValue={[];[]}
      settings: InputPortMap=u0,u1
  Fulfillment_Shipment : PMIOPort  Port=1  Side=Right
  Customer_Procurement_Order : PMIOPort  Port=2  Side=Right
  wires:
  Get_Order_Attributes/2 -> Set_Shipment_Attributes/1
  Get_Order_Attributes/1 -> Set_Shipment_Attributes/2
  connections:
  Customer_Procurement_Order/RConn1 -- Get_Order_Attributes/LConn1
  Fulfillment_Shipment/RConn1 -- Set_Shipment_Attributes/RConn1
  N-Server/RConn1 -- Set_Shipment_Attributes/LConn1
  FIFO Queue/RConn1 -- N-Server/LConn1
  FIFO Queue/LConn1 -- Get_Order_Attributes/RConn1

== system HubDepotModel/Supplier_2/Supplier ==
  FIFO Queue : FIFOQueue
  Get_Order_Attributes : GetAttribute  AttributeName=Order_Quantity|Component  AttributeMissing=Error|Error  AttributeDefaultValue=1|1  AttributeTreatAsVector=1|1  AttributeSendTiming=After entity departure|After entity departure  EvaluatedDefaultAttributeValue={[];[]}
      settings: OutputPortMap=o1,o2
  N-Server : NServer  NumberOfServers=inf  ServiceTime=0
  Set_Shipment_Attributes : SetAttribute  AttributeName=Component|Shipment_Quantity  AttributeFrom=Signal port|Signal port  AttributeValue=1|3  AttributeTreatAsVector=1|1  EvaluatedAttributeValue={[];[]}
      settings: InputPortMap=u0,u1
  Fulfillment_Shipment : PMIOPort  Port=1  Side=Right
  Customer_Procurement_Order : PMIOPort  Port=2  Side=Right
  wires:
  Get_Order_Attributes/2 -> Set_Shipment_Attributes/1
  Get_Order_Attributes/1 -> Set_Shipment_Attributes/2
  connections:
  Customer_Procurement_Order/RConn1 -- Get_Order_Attributes/LConn1
  Fulfillment_Shipment/RConn1 -- Set_Shipment_Attributes/RConn1
  N-Server/RConn1 -- Set_Shipment_Attributes/LConn1
  FIFO Queue/RConn1 -- N-Server/LConn1
  FIFO Queue/LConn1 -- Get_Order_Attributes/RConn1

== system HubDepotModel/Depot_1/Storage_Subsystem/<<DELIVER>>Deliver_Stocked_Product ==
  Deliver_Stocked_Product_CONTROL : Subsystem
  sD1.10_Pack_Order_PLANT : Subsystem
  sD1.11_Load_Order_PLANT : Subsystem
  sD1.2_Receive_Order_PLANT : Subsystem
  sD1.4_Consolidate_Orders_PLANT : Subsystem
  sD1.9_Pick_Order_PLANT : Subsystem
  Inventory_IN : PMIOPort  Port=1  Side=Left
  Inventory_OUT : PMIOPort  Port=2  Side=Right
  Customer_Procurement_Order : PMIOPort  Port=3  Side=Left
  Fulfillment_Shipment : PMIOPort  Port=4  Side=Right
  Replenishment_Signal : PMIOPort  Port=5  Side=Right
  connections:
  sD1.4_Consolidate_Orders_PLANT/RConn1 -- sD1.9_Pick_Order_PLANT/LConn1
  sD1.2_Receive_Order_PLANT/RConn1 -- sD1.4_Consolidate_Orders_PLANT/LConn1
  Deliver_Stocked_Product_CONTROL/RConn2 -- Inventory_OUT/RConn1
  Deliver_Stocked_Product_CONTROL/RConn1 -- Replenishment_Signal/RConn1
  Deliver_Stocked_Product_CONTROL/LConn1 -- Inventory_IN/RConn1
  sD1.9_Pick_Order_PLANT/RConn1 -- Deliver_Stocked_Product_CONTROL/LConn2
  sD1.11_Load_Order_PLANT/RConn1 -- Fulfillment_Shipment/RConn1
  sD1.10_Pack_Order_PLANT/RConn1 -- sD1.11_Load_Order_PLANT/LConn1
  sD1.9_Pick_Order_PLANT/RConn2 -- sD1.10_Pack_Order_PLANT/LConn1
  Customer_Procurement_Order/RConn1 -- sD1.2_Receive_Order_PLANT/LConn1

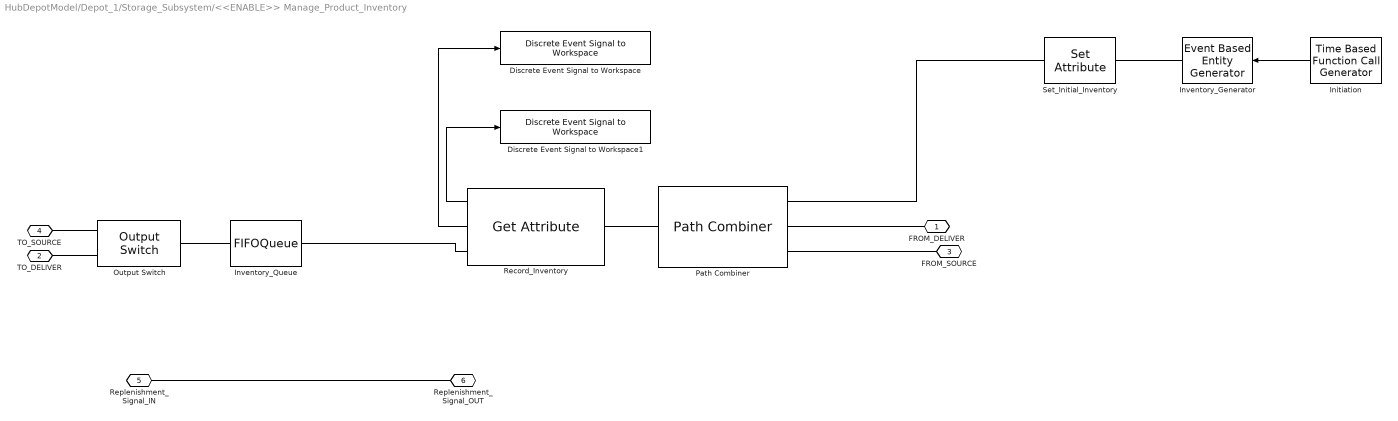
== system HubDepotModel/Depot_1/Storage_Subsystem/<<ENABLE>> Manage_Product_Inventory ==
  Discrete Event Signal to Workspace : simeventslib/SimEvents Sinks/Discrete Event Signal to Workspace  VariableName=Inventory_Position_Depot_1  SaveFormat=Structure With Time  isMonitorOnly=off  isRecordIC=off
  Discrete Event Signal to Workspace1 : simeventslib/SimEvents Sinks/Discrete Event Signal to Workspace  VariableName=Net_Inventory_Depot_1  SaveFormat=Structure With Time  isMonitorOnly=off  isRecordIC=off
  Initiation : TimeBasedFunctionCallGenerator  EventGenerationMode=Only at simulation start  EventPriority=1
  Inventory_Generator : EventBasedEntityGenerator  GenerateEntitiesUpon=Function call from port fcn  SpecifyEventPriority=on  PriorityEntityGeneration=1  AllowBlocking=off  EntityType=Standard
  Inventory_Queue : FIFOQueue
  Output Switch : OutputSwitch  NumberOutputPorts=2
  Path Combiner : PathCombiner
  Record_Inventory : GetAttribute  AttributeName=Net_Inventory|Inventory_Position  AttributeMissing=Error|Error  AttributeDefaultValue=1|1  AttributeTreatAsVector=1|1  AttributeSendTiming=After entity departure|After entity departure  EvaluatedDefaultAttributeValue={[];[]}
      settings: OutputPortMap=o1,o2
  Set_Initial_Inventory : SetAttribute  AttributeName=Net_Inventory|Inventory_Position|Reorder_Point|Reorder_Quantity  AttributeFrom=Dialog|Dialog|Dialog|Dialog  AttributeValue=[11 13]|[11 13]|[10 10]|[5 5]  AttributeTreatAsVector=1|1|1|1  EvaluatedAttributeValue={[11 13];[11 13];[10 10];[5 5]}
  FROM_DELIVER : PMIOPort  Port=1  Side=Left
  TO_DELIVER : PMIOPort  Port=2  Side=Right
  FROM_SOURCE : PMIOPort  Port=3  Side=Left
  TO_SOURCE : PMIOPort  Port=4  Side=Right
  Replenishment_Signal_IN : PMIOPort  Port=5  Side=Left
  Replenishment_Signal_OUT : PMIOPort  Port=6  Side=Right
  wires:
  Record_Inventory/2 -> Discrete Event Signal to Workspace/1
  Initiation/1 -> Inventory_Generator/1
  Record_Inventory/1 -> Discrete Event Signal to Workspace1/1
  connections:
  Set_Initial_Inventory/RConn1 -- Path Combiner/LConn1
  Replenishment_Signal_IN/RConn1 -- Replenishment_Signal_OUT/RConn1
  TO_SOURCE/RConn1 -- Output Switch/RConn1
  TO_DELIVER/RConn1 -- Output Switch/RConn2
  FROM_SOURCE/RConn1 -- Path Combiner/LConn3
  FROM_DELIVER/RConn1 -- Path Combiner/LConn2
  Record_Inventory/LConn1 -- Path Combiner/RConn1
  Output Switch/LConn1 -- Inventory_Queue/RConn1
  Record_Inventory/RConn1 -- Inventory_Queue/LConn1
  Set_Initial_Inventory/LConn1 -- Inventory_Generator/RConn1

== system HubDepotModel/Depot_1/Storage_Subsystem/<<SOURCE>> Source_Stocked_Product ==
  Output Switch : OutputSwitch  NumberOutputPorts=2
  Path Combiner : PathCombiner  NumberInputPorts=2
  Schedule_Product_Deliveries_CONTROL : Subsystem
  Transfer_Product_CONTROL : Subsystem
  sS1.1_Schedule_Product_Deliveries_PLANT : Subsystem
  sS1.2_Receive_Product_PLANT : Subsystem
  sS1.3_Transfer_Product_PLANT : Subsystem
  sS1.3_Verify_Product_PLANT : Subsystem
  Inventory_IN : PMIOPort  Port=1  Side=Left
  Inventory_OUT : PMIOPort  Port=2  Side=Right
  Replenishment_Shipment : PMIOPort  Port=3  Side=Left
  Replenishment_Signal : PMIOPort  Port=4  Side=Left
  Procurement_Order : PMIOPort  Port=5  Side=Right
  wires:
  Schedule_Product_Deliveries_CONTROL/3(Reorder_Signal) -> sS1.1_Schedule_Product_Deliveries_PLANT/3(Reorder_Signal)
  Schedule_Product_Deliveries_CONTROL/1(Component) -> sS1.1_Schedule_Product_Deliveries_PLANT/1(Component)
  Schedule_Product_Deliveries_CONTROL/2(Reorder_Quantity) -> sS1.1_Schedule_Product_Deliveries_PLANT/2(Reorder_Quantity)
  connections:
  Replenishment_Signal/RConn1 -- Schedule_Product_Deliveries_CONTROL/LConn2
  Path Combiner/LConn1 -- Schedule_Product_Deliveries_CONTROL/RConn1
  Path Combiner/LConn2 -- Transfer_Product_CONTROL/RConn1
  Path Combiner/RConn1 -- Inventory_OUT/RConn1
  Output Switch/RConn2 -- Transfer_Product_CONTROL/LConn1
  Output Switch/RConn1 -- Schedule_Product_Deliveries_CONTROL/LConn1
  Inventory_IN/RConn1 -- Output Switch/LConn1
  sS1.1_Schedule_Product_Deliveries_PLANT/RConn1 -- Procurement_Order/RConn1
  sS1.3_Transfer_Product_PLANT/RConn1 -- Transfer_Product_CONTROL/LConn2
  sS1.3_Verify_Product_PLANT/RConn1 -- sS1.3_Transfer_Product_PLANT/LConn1
  sS1.2_Receive_Product_PLANT/RConn1 -- sS1.3_Verify_Product_PLANT/LConn1
  Replenishment_Shipment/RConn1 -- sS1.2_Receive_Product_PLANT/LConn1

== system HubDepotModel/Depot_2/Storage_Subsystem/<<DELIVER>>Deliver_Stocked_Product ==
  Deliver_Stocked_Product_CONTROL : Subsystem
  sD1.10_Pack_Order_PLANT : Subsystem
  sD1.11_Load_Order_PLANT : Subsystem
  sD1.2_Receive_Order_PLANT : Subsystem
  sD1.4_Consolidate_Orders_PLANT : Subsystem
  sD1.9_Pick_Order_PLANT : Subsystem
  Inventory_IN : PMIOPort  Port=1  Side=Left
  Inventory_OUT : PMIOPort  Port=2  Side=Right
  Customer_Procurement_Order : PMIOPort  Port=3  Side=Left
  Fulfillment_Shipment : PMIOPort  Port=4  Side=Right
  Replenishment_Signal : PMIOPort  Port=5  Side=Right
  connections:
  sD1.4_Consolidate_Orders_PLANT/RConn1 -- sD1.9_Pick_Order_PLANT/LConn1
  sD1.2_Receive_Order_PLANT/RConn1 -- sD1.4_Consolidate_Orders_PLANT/LConn1
  Deliver_Stocked_Product_CONTROL/RConn2 -- Inventory_OUT/RConn1
  Deliver_Stocked_Product_CONTROL/RConn1 -- Replenishment_Signal/RConn1
  Deliver_Stocked_Product_CONTROL/LConn1 -- Inventory_IN/RConn1
  sD1.9_Pick_Order_PLANT/RConn1 -- Deliver_Stocked_Product_CONTROL/LConn2
  sD1.11_Load_Order_PLANT/RConn1 -- Fulfillment_Shipment/RConn1
  sD1.10_Pack_Order_PLANT/RConn1 -- sD1.11_Load_Order_PLANT/LConn1
  sD1.9_Pick_Order_PLANT/RConn2 -- sD1.10_Pack_Order_PLANT/LConn1
  Customer_Procurement_Order/RConn1 -- sD1.2_Receive_Order_PLANT/LConn1

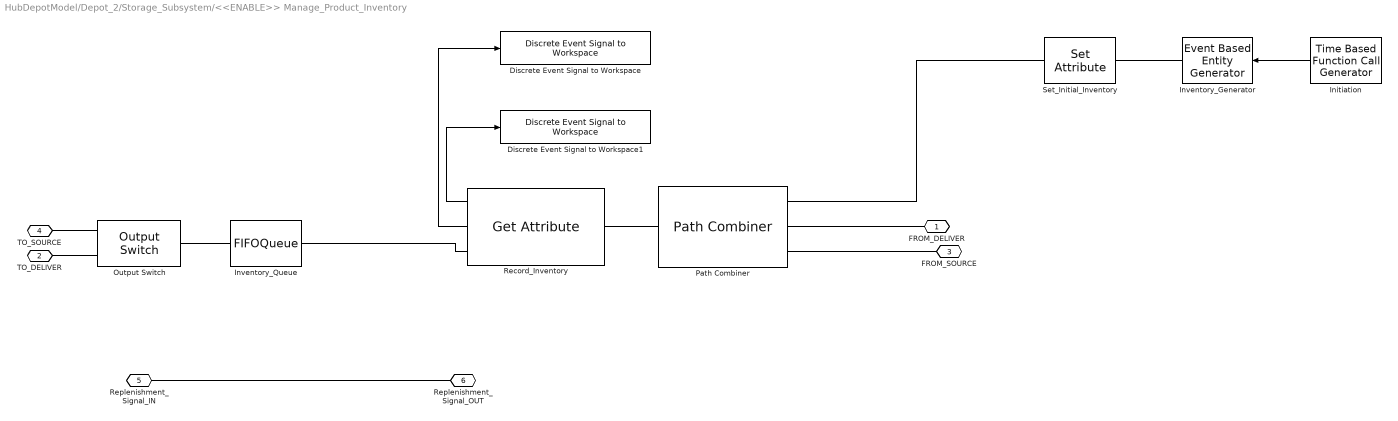
== system HubDepotModel/Depot_2/Storage_Subsystem/<<ENABLE>> Manage_Product_Inventory ==
  Discrete Event Signal to Workspace : simeventslib/SimEvents Sinks/Discrete Event Signal to Workspace  VariableName=Inventory_Position_Depot_1  SaveFormat=Structure With Time  isMonitorOnly=off  isRecordIC=off
  Discrete Event Signal to Workspace1 : simeventslib/SimEvents Sinks/Discrete Event Signal to Workspace  VariableName=Net_Inventory_Depot_1  SaveFormat=Structure With Time  isMonitorOnly=off  isRecordIC=off
  Initiation : TimeBasedFunctionCallGenerator  EventGenerationMode=Only at simulation start  EventPriority=1
  Inventory_Generator : EventBasedEntityGenerator  GenerateEntitiesUpon=Function call from port fcn  SpecifyEventPriority=on  PriorityEntityGeneration=1  AllowBlocking=off  EntityType=Standard
  Inventory_Queue : FIFOQueue
  Output Switch : OutputSwitch  NumberOutputPorts=2
  Path Combiner : PathCombiner
  Record_Inventory : GetAttribute  AttributeName=Net_Inventory|Inventory_Position  AttributeMissing=Error|Error  AttributeDefaultValue=1|1  AttributeTreatAsVector=1|1  AttributeSendTiming=After entity departure|After entity departure  EvaluatedDefaultAttributeValue={[];[]}
      settings: OutputPortMap=o1,o2
  Set_Initial_Inventory : SetAttribute  AttributeName=Net_Inventory|Inventory_Position|Reorder_Point|Reorder_Quantity  AttributeFrom=Dialog|Dialog|Dialog|Dialog  AttributeValue=[11 13]|[11 13]|[10 10]|[5 5]  AttributeTreatAsVector=1|1|1|1  EvaluatedAttributeValue={[11 13];[11 13];[10 10];[5 5]}
  FROM_DELIVER : PMIOPort  Port=1  Side=Left
  TO_DELIVER : PMIOPort  Port=2  Side=Right
  FROM_SOURCE : PMIOPort  Port=3  Side=Left
  TO_SOURCE : PMIOPort  Port=4  Side=Right
  Replenishment_Signal_IN : PMIOPort  Port=5  Side=Left
  Replenishment_Signal_OUT : PMIOPort  Port=6  Side=Right
  wires:
  Record_Inventory/2 -> Discrete Event Signal to Workspace/1
  Initiation/1 -> Inventory_Generator/1
  Record_Inventory/1 -> Discrete Event Signal to Workspace1/1
  connections:
  Set_Initial_Inventory/RConn1 -- Path Combiner/LConn1
  Replenishment_Signal_IN/RConn1 -- Replenishment_Signal_OUT/RConn1
  TO_SOURCE/RConn1 -- Output Switch/RConn1
  TO_DELIVER/RConn1 -- Output Switch/RConn2
  FROM_SOURCE/RConn1 -- Path Combiner/LConn3
  FROM_DELIVER/RConn1 -- Path Combiner/LConn2
  Record_Inventory/LConn1 -- Path Combiner/RConn1
  Output Switch/LConn1 -- Inventory_Queue/RConn1
  Record_Inventory/RConn1 -- Inventory_Queue/LConn1
  Set_Initial_Inventory/LConn1 -- Inventory_Generator/RConn1

== system HubDepotModel/Depot_2/Storage_Subsystem/<<SOURCE>> Source_Stocked_Product ==
  Output Switch : OutputSwitch  NumberOutputPorts=2
  Path Combiner : PathCombiner  NumberInputPorts=2
  Schedule_Product_Deliveries_CONTROL : Subsystem
  Transfer_Product_CONTROL : Subsystem
  sS1.1_Schedule_Product_Deliveries_PLANT : Subsystem
  sS1.2_Receive_Product_PLANT : Subsystem
  sS1.3_Transfer_Product_PLANT : Subsystem
  sS1.3_Verify_Product_PLANT : Subsystem
  Inventory_IN : PMIOPort  Port=1  Side=Left
  Inventory_OUT : PMIOPort  Port=2  Side=Right
  Replenishment_Shipment : PMIOPort  Port=3  Side=Left
  Replenishment_Signal : PMIOPort  Port=4  Side=Left
  Procurement_Order : PMIOPort  Port=5  Side=Right
  wires:
  Schedule_Product_Deliveries_CONTROL/3(Reorder_Signal) -> sS1.1_Schedule_Product_Deliveries_PLANT/3(Reorder_Signal)
  Schedule_Product_Deliveries_CONTROL/1(Component) -> sS1.1_Schedule_Product_Deliveries_PLANT/1(Component)
  Schedule_Product_Deliveries_CONTROL/2(Reorder_Quantity) -> sS1.1_Schedule_Product_Deliveries_PLANT/2(Reorder_Quantity)
  connections:
  Replenishment_Signal/RConn1 -- Schedule_Product_Deliveries_CONTROL/LConn2
  Path Combiner/LConn1 -- Schedule_Product_Deliveries_CONTROL/RConn1
  Path Combiner/LConn2 -- Transfer_Product_CONTROL/RConn1
  Path Combiner/RConn1 -- Inventory_OUT/RConn1
  Output Switch/RConn2 -- Transfer_Product_CONTROL/LConn1
  Output Switch/RConn1 -- Schedule_Product_Deliveries_CONTROL/LConn1
  Inventory_IN/RConn1 -- Output Switch/LConn1
  sS1.1_Schedule_Product_Deliveries_PLANT/RConn1 -- Procurement_Order/RConn1
  sS1.3_Transfer_Product_PLANT/RConn1 -- Transfer_Product_CONTROL/LConn2
  sS1.3_Verify_Product_PLANT/RConn1 -- sS1.3_Transfer_Product_PLANT/LConn1
  sS1.2_Receive_Product_PLANT/RConn1 -- sS1.3_Verify_Product_PLANT/LConn1
  Replenishment_Shipment/RConn1 -- sS1.2_Receive_Product_PLANT/LConn1

== system HubDepotModel/Depot_3/Storage_Subsystem/<<DELIVER>>Deliver_Stocked_Product ==
  Deliver_Stocked_Product_CONTROL : Subsystem
  sD1.10_Pack_Order_PLANT : Subsystem
  sD1.11_Load_Order_PLANT : Subsystem
  sD1.2_Receive_Order_PLANT : Subsystem
  sD1.4_Consolidate_Orders_PLANT : Subsystem
  sD1.9_Pick_Order_PLANT : Subsystem
  Inventory_IN : PMIOPort  Port=1  Side=Left
  Inventory_OUT : PMIOPort  Port=2  Side=Right
  Customer_Procurement_Order : PMIOPort  Port=3  Side=Left
  Fulfillment_Shipment : PMIOPort  Port=4  Side=Right
  Replenishment_Signal : PMIOPort  Port=5  Side=Right
  connections:
  sD1.4_Consolidate_Orders_PLANT/RConn1 -- sD1.9_Pick_Order_PLANT/LConn1
  sD1.2_Receive_Order_PLANT/RConn1 -- sD1.4_Consolidate_Orders_PLANT/LConn1
  Deliver_Stocked_Product_CONTROL/RConn2 -- Inventory_OUT/RConn1
  Deliver_Stocked_Product_CONTROL/RConn1 -- Replenishment_Signal/RConn1
  Deliver_Stocked_Product_CONTROL/LConn1 -- Inventory_IN/RConn1
  sD1.9_Pick_Order_PLANT/RConn1 -- Deliver_Stocked_Product_CONTROL/LConn2
  sD1.11_Load_Order_PLANT/RConn1 -- Fulfillment_Shipment/RConn1
  sD1.10_Pack_Order_PLANT/RConn1 -- sD1.11_Load_Order_PLANT/LConn1
  sD1.9_Pick_Order_PLANT/RConn2 -- sD1.10_Pack_Order_PLANT/LConn1
  Customer_Procurement_Order/RConn1 -- sD1.2_Receive_Order_PLANT/LConn1

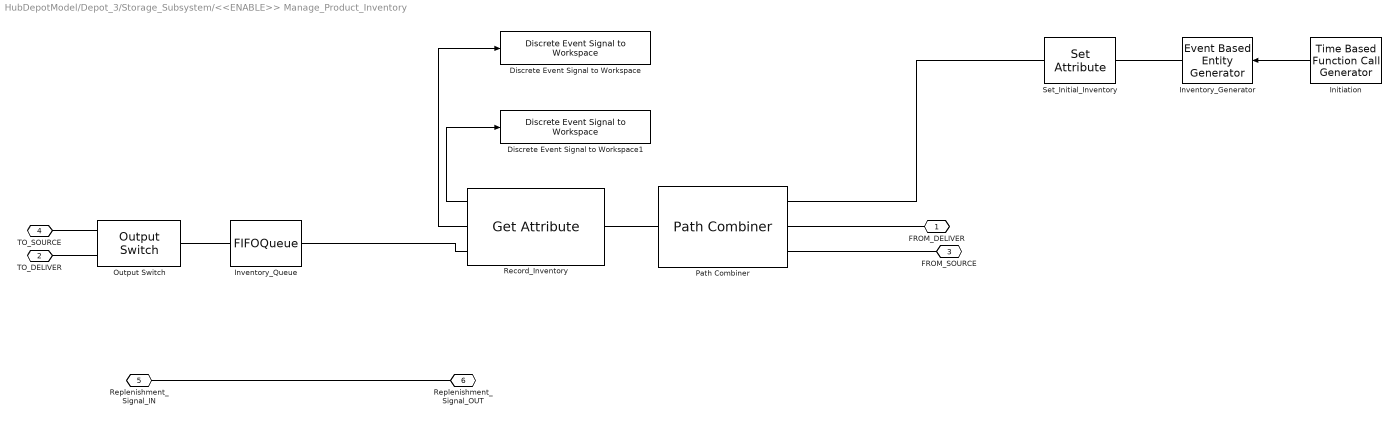
== system HubDepotModel/Depot_3/Storage_Subsystem/<<ENABLE>> Manage_Product_Inventory ==
  Discrete Event Signal to Workspace : simeventslib/SimEvents Sinks/Discrete Event Signal to Workspace  VariableName=Inventory_Position_Depot_1  SaveFormat=Structure With Time  isMonitorOnly=off  isRecordIC=off
  Discrete Event Signal to Workspace1 : simeventslib/SimEvents Sinks/Discrete Event Signal to Workspace  VariableName=Net_Inventory_Depot_1  SaveFormat=Structure With Time  isMonitorOnly=off  isRecordIC=off
  Initiation : TimeBasedFunctionCallGenerator  EventGenerationMode=Only at simulation start  EventPriority=1
  Inventory_Generator : EventBasedEntityGenerator  GenerateEntitiesUpon=Function call from port fcn  SpecifyEventPriority=on  PriorityEntityGeneration=1  AllowBlocking=off  EntityType=Standard
  Inventory_Queue : FIFOQueue
  Output Switch : OutputSwitch  NumberOutputPorts=2
  Path Combiner : PathCombiner
  Record_Inventory : GetAttribute  AttributeName=Net_Inventory|Inventory_Position  AttributeMissing=Error|Error  AttributeDefaultValue=1|1  AttributeTreatAsVector=1|1  AttributeSendTiming=After entity departure|After entity departure  EvaluatedDefaultAttributeValue={[];[]}
      settings: OutputPortMap=o1,o2
  Set_Initial_Inventory : SetAttribute  AttributeName=Net_Inventory|Inventory_Position|Reorder_Point|Reorder_Quantity  AttributeFrom=Dialog|Dialog|Dialog|Dialog  AttributeValue=[11 13]|[11 13]|[10 10]|[5 5]  AttributeTreatAsVector=1|1|1|1  EvaluatedAttributeValue={[11 13];[11 13];[10 10];[5 5]}
  FROM_DELIVER : PMIOPort  Port=1  Side=Left
  TO_DELIVER : PMIOPort  Port=2  Side=Right
  FROM_SOURCE : PMIOPort  Port=3  Side=Left
  TO_SOURCE : PMIOPort  Port=4  Side=Right
  Replenishment_Signal_IN : PMIOPort  Port=5  Side=Left
  Replenishment_Signal_OUT : PMIOPort  Port=6  Side=Right
  wires:
  Record_Inventory/2 -> Discrete Event Signal to Workspace/1
  Initiation/1 -> Inventory_Generator/1
  Record_Inventory/1 -> Discrete Event Signal to Workspace1/1
  connections:
  Set_Initial_Inventory/RConn1 -- Path Combiner/LConn1
  Replenishment_Signal_IN/RConn1 -- Replenishment_Signal_OUT/RConn1
  TO_SOURCE/RConn1 -- Output Switch/RConn1
  TO_DELIVER/RConn1 -- Output Switch/RConn2
  FROM_SOURCE/RConn1 -- Path Combiner/LConn3
  FROM_DELIVER/RConn1 -- Path Combiner/LConn2
  Record_Inventory/LConn1 -- Path Combiner/RConn1
  Output Switch/LConn1 -- Inventory_Queue/RConn1
  Record_Inventory/RConn1 -- Inventory_Queue/LConn1
  Set_Initial_Inventory/LConn1 -- Inventory_Generator/RConn1
